simulink library "Vehicle_Visualization"  (R2026a)
settings: Solver=VariableStepAuto
undefined symbols (not defined in the file): unreal_timeseries
libraries: $bdroot x9, sm_car_lib x2, vehdynlibviscommon x1
Description:
  | Copyright 2018-2026 The MathWorks, Inc.
settings Model: Creator=smiller  LastModifiedBy=smiller

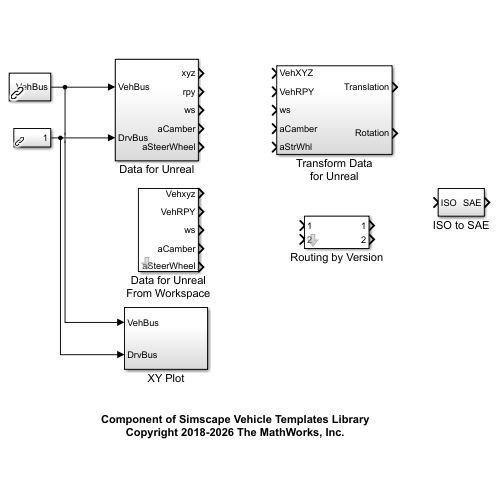
[thumbnail: Simulink's stored preview of the top-level diagram]
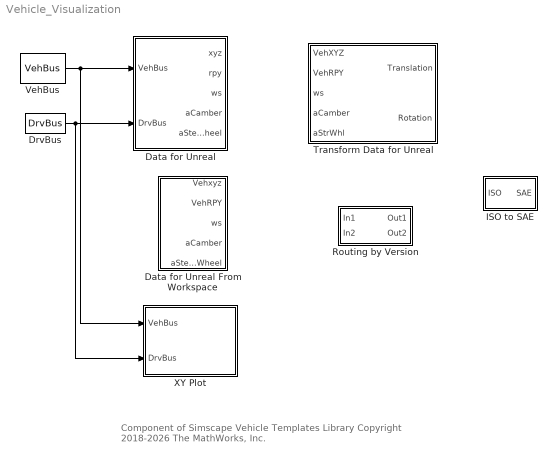
== system Vehicle_Visualization ==
  note: Component of Simscape Vehicle Templates Library
      | Copyright 2018-2026 The MathWorks, Inc.
  Data for Unreal : Subsystem
  Data for Unreal From Workspace : Subsystem  mask(Timeseries data for replay){unreal_data=unreal_timeseries}
      mask prompts: unreal_data "Unreal Time Series"
      mask help: Unpacks timeseries data for use with Vehicle Dynamics Blockset connection to Unreal visualization.
  DrvBus : sm_car_lib/Inputs/DrvBus  SystemSampleTime=-1  VariantActivationTime=update diagram  EmptyChoice=off  PassThrough=off  PassThroughVariantControl=(default)  EmptyChoiceVariantControl=(default)  AllowFlexibleInterface=on  Latency=0  AutoFrameSizeCalculation=off
  ISO to SAE : Subsystem
  Routing by Version : Subsystem  mask(Swap Inputs based on MATLAB Release){post_19a=1}
      mask prompts: post_19a "After R19a?"
      mask help: Unreal Engine inputs of Pitch and Roll were swapped for Wheel Inputs in R2019b. This block swaps order of two inputs based on MATLAB release.
      mask init:
      | if(verLessThan('matlab','9.7'))
      |     set_param(gcb,'post_19a','1');
      | else
      |     set_param(gcb,'post_19a','-1');
      | end
  Transform Data for Unreal : Subsystem
  VehBus : sm_car_lib/Outputs/VehBus  SystemSampleTime=-1  VariantActivationTime=update diagram  EmptyChoice=off  PassThrough=off  PassThroughVariantControl=(default)  EmptyChoiceVariantControl=(default)  AllowFlexibleInterface=on  Latency=0  AutoFrameSizeCalculation=off
  XY Plot : Subsystem
  wires:
  VehBus/1 -> Data for Unreal/1(VehBus), XY Plot/1(VehBus)
  DrvBus/1 -> Data for Unreal/2(DrvBus), XY Plot/2(DrvBus)

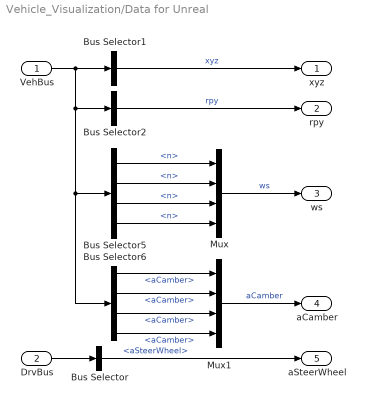
== system Vehicle_Visualization/Data for Unreal ==
  VehBus : Inport
  DrvBus : Inport  Port=2
  Bus Selector : BusSelector  OutputSignals=aSteerWheel
  Bus Selector1 : BusSelector  OutputSignals=World.x,World.y,World.z  OutputAsBus=on
  Bus Selector2 : BusSelector  OutputSignals=World.aRoll,World.aPitch,World.aYaw  OutputAsBus=on
  Bus Selector5 : BusSelector  OutputSignals=Chassis.WhlL1.n,Chassis.WhlR1.n,Chassis.WhlL2.n,Chassis.WhlR2.n
  Bus Selector6 : BusSelector  OutputSignals=Chassis.WhlL1.aCamber,Chassis.WhlR1.aCamber,Chassis.WhlL2.aCamber,Chassis.WhlR2.aCamber
  Mux : Mux
  Mux1 : Mux
  xyz : Outport  VectorParamsAs1DForOutWhenUnconnected=off
  rpy : Outport  Port=2  VectorParamsAs1DForOutWhenUnconnected=off
  ws : Outport  Port=3  VectorParamsAs1DForOutWhenUnconnected=off
  aCamber : Outport  Port=4  VectorParamsAs1DForOutWhenUnconnected=off
  aSteerWheel : Outport  Port=5  VectorParamsAs1DForOutWhenUnconnected=off
  wires:
  Bus Selector5/3 -> Mux/3  "<n>"
  Bus Selector1/1 -> xyz/1  "xyz"
  Mux1/1 -> aCamber/1  "aCamber"
  VehBus/1 -> Bus Selector6/1, Bus Selector5/1, Bus Selector2/1, Bus Selector1/1
  DrvBus/1 -> Bus Selector/1
  Bus Selector5/4 -> Mux/4  "<n>"
  Bus Selector5/2 -> Mux/2  "<n>"
  Bus Selector5/1 -> Mux/1  "<n>"
  Bus Selector6/1 -> Mux1/1  "<aCamber>"
  Bus Selector2/1 -> rpy/1  "rpy"
  Mux/1 -> ws/1  "ws"
  Bus Selector6/2 -> Mux1/2  "<aCamber>"
  Bus Selector6/3 -> Mux1/3  "<aCamber>"
  Bus Selector6/4 -> Mux1/4  "<aCamber>"
  Bus Selector/1 -> aSteerWheel/1  "<aSteerWheel>"

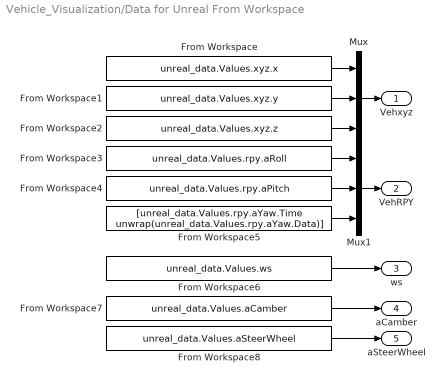
== system Vehicle_Visualization/Data for Unreal From Workspace ==
  From Workspace : FromWorkspace  VariableName=unreal_data.Values.xyz.x
  From Workspace1 : FromWorkspace  VariableName=unreal_data.Values.xyz.y
  From Workspace2 : FromWorkspace  VariableName=unreal_data.Values.xyz.z
  From Workspace3 : FromWorkspace  VariableName=unreal_data.Values.rpy.aRoll
  From Workspace4 : FromWorkspace  VariableName=unreal_data.Values.rpy.aPitch
  From Workspace5 : FromWorkspace  VariableName=[unreal_data.Values.rpy.aYaw.Time unwrap(unreal_data.Values.rpy.aYaw.Data)]
  From Workspace6 : FromWorkspace  VariableName=unreal_data.Values.ws
  From Workspace7 : FromWorkspace  VariableName=unreal_data.Values.aCamber
  From Workspace8 : FromWorkspace  VariableName=unreal_data.Values.aSteerWheel
  Mux : Mux  Inputs=3
  Mux1 : Mux  Inputs=3
  Vehxyz : Outport  VectorParamsAs1DForOutWhenUnconnected=off
  VehRPY : Outport  Port=2  VectorParamsAs1DForOutWhenUnconnected=off
  ws : Outport  Port=3  VectorParamsAs1DForOutWhenUnconnected=off
  aCamber : Outport  Port=4  VectorParamsAs1DForOutWhenUnconnected=off
  aSteerWheel : Outport  Port=5  VectorParamsAs1DForOutWhenUnconnected=off
  wires:
  From Workspace7/1 -> aCamber/1
  From Workspace8/1 -> aSteerWheel/1
  Mux1/1 -> VehRPY/1
  From Workspace3/1 -> Mux1/1
  From Workspace1/1 -> Mux/2
  From Workspace2/1 -> Mux/3
  From Workspace5/1 -> Mux1/3
  From Workspace4/1 -> Mux1/2
  From Workspace6/1 -> ws/1
  Mux/1 -> Vehxyz/1
  From Workspace/1 -> Mux/1

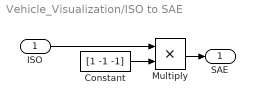
== system Vehicle_Visualization/ISO to SAE ==
  ISO : Inport
  Constant : Constant  Value=[1 -1 -1]
  Multiply : Product
  SAE : Outport  VectorParamsAs1DForOutWhenUnconnected=off
  wires:
  Constant/1 -> Multiply/2
  ISO/1 -> Multiply/1
  Multiply/1 -> SAE/1

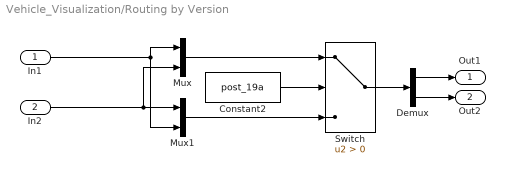
== system Vehicle_Visualization/Routing by Version ==
  In1 : Inport
  In2 : Inport  Port=2
  Constant2 : Constant  Value=post_19a
  Demux : Demux  Outputs=2
  Mux : Mux  Inputs=2
  Mux1 : Mux  Inputs=2
  Switch : Switch  Criteria=u2 > Threshold  SaturateOnIntegerOverflow=off  InputSameDT=off
  Out1 : Outport  VectorParamsAs1DForOutWhenUnconnected=off
  Out2 : Outport  Port=2  VectorParamsAs1DForOutWhenUnconnected=off
  wires:
  Demux/2 -> Out2/1
  Demux/1 -> Out1/1
  Mux1/1 -> Switch/3
  Constant2/1 -> Switch/2
  In1/1 -> Mux1/2, Mux/1
  In2/1 -> Mux1/1, Mux/2
  Mux/1 -> Switch/1
  Switch/1 -> Demux/1

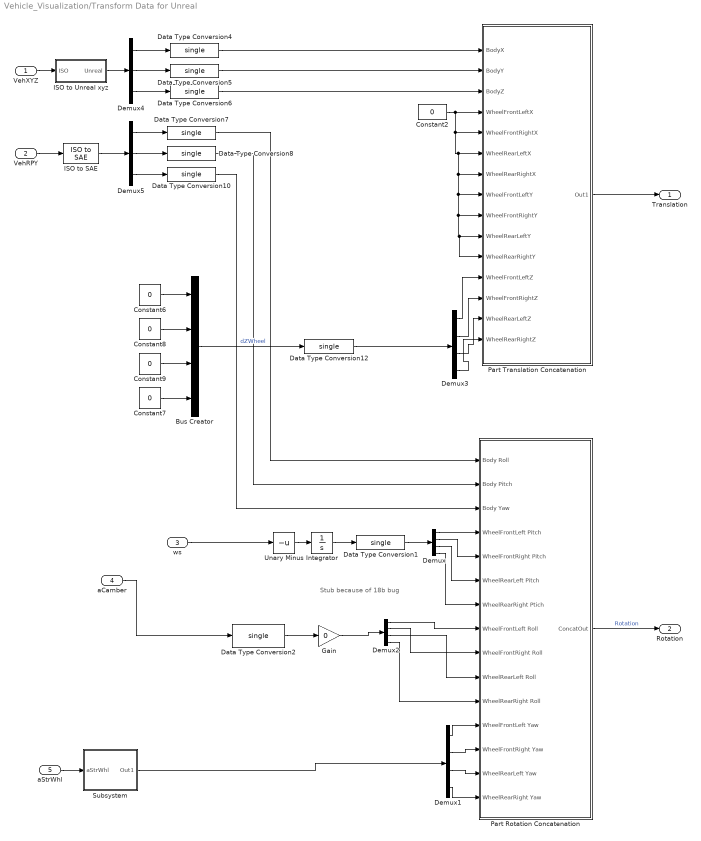
== system Vehicle_Visualization/Transform Data for Unreal ==
  note: Stub because of 18b bug
  VehXYZ : Inport
  VehRPY : Inport  Port=2
  ws : Inport  Port=3
  aCamber : Inport  Port=4
  aStrWhl : Inport  Port=5
  Bus Creator : BusCreator  Inputs=4
  Constant2 : Constant  Value=0  OutDataTypeStr=single
  Constant{6..9} (4 alike) : Constant  Value=0
  Data Type Conversion{1..2,4..8,10,12} (9 alike) : DataTypeConversion  OutDataTypeStr=single  SaturateOnIntegerOverflow=off  RndMeth=Floor
  Demux{,1..3} (4 alike) : Demux
  Demux4 : Demux  Outputs=3
  Demux5 : Demux  Outputs=3
  Gain : Gain  Gain=0
  "ISO to SAE " : $bdroot/ISO to SAE  SystemSampleTime=-1  VariantActivationTime=update diagram  EmptyChoice=off  PassThrough=off  PassThroughVariantControl=(default)  EmptyChoiceVariantControl=(default)  AllowFlexibleInterface=on  Latency=0  AutoFrameSizeCalculation=off
  ISO to Unreal xyz : Subsystem
  Integrator : Integrator
  Part Rotation Concatenation : Subsystem
  Part Translation Concatenation : Subsystem
  Subsystem : Subsystem
  Unary Minus : UnaryMinus
  Translation : Outport  VectorParamsAs1DForOutWhenUnconnected=off
  Rotation : Outport  Port=2  VectorParamsAs1DForOutWhenUnconnected=off
  wires:
  aStrWhl/1 -> Subsystem/1(aStrWhl)
  Part Translation Concatenation/1(Out1) -> Translation/1
  aCamber/1 -> Data Type Conversion2/1
  ws/1 -> Unary Minus/1
  VehRPY/1 -> "ISO to SAE "/1
  "ISO to SAE "/1 -> Demux5/1
  Demux4/2 -> Data Type Conversion5/1
  Demux4/1 -> Data Type Conversion4/1
  ISO to Unreal xyz/1(Unreal) -> Demux4/1
  VehXYZ/1 -> ISO to Unreal xyz/1(ISO)
  Part Rotation Concatenation/1(ConcatOut) -> Rotation/1  "Rotation"
  Subsystem/1(Out1) -> Demux1/1
  Data Type Conversion10/1 -> Part Rotation Concatenation/3(Body Yaw)
  Demux/1 -> Part Rotation Concatenation/4(WheelFrontLeft Pitch)
  Integrator/1 -> Data Type Conversion1/1
  Data Type Conversion2/1 -> Gain/1
  Demux/3 -> Part Rotation Concatenation/6(WheelRearLeft Pitch)
  Demux2/3 -> Part Rotation Concatenation/10(WheelRearLeft Roll)
  Constant7/1 -> Bus Creator/4
  Data Type Conversion6/1 -> Part Translation Concatenation/3(BodyZ)
  Data Type Conversion8/1 -> Part Rotation Concatenation/2(Body Pitch)
  Demux2/1 -> Part Rotation Concatenation/8(WheelFrontLeft Roll)
  Demux2/4 -> Part Rotation Concatenation/11(WheelRearRight Roll)
  Constant6/1 -> Bus Creator/1
  Demux1/2 -> Part Rotation Concatenation/13(WheelFrontRight Yaw)
  Data Type Conversion5/1 -> Part Translation Concatenation/2(BodyY)
  Demux/4 -> Part Rotation Concatenation/7(WheelRearRight Ptich)
  Unary Minus/1 -> Integrator/1
  Constant8/1 -> Bus Creator/2
  Demux1/4 -> Part Rotation Concatenation/15(WheelRearRight Yaw)
  Data Type Conversion1/1 -> Demux/1
  Demux5/1 -> Data Type Conversion7/1
  Demux2/2 -> Part Rotation Concatenation/9(WheelFrontRight Roll)
  Demux1/1 -> Part Rotation Concatenation/12(WheelFrontLeft Yaw)
  Gain/1 -> Demux2/1
  Demux4/3 -> Data Type Conversion6/1
  Data Type Conversion4/1 -> Part Translation Concatenation/1(BodyX)
  Demux5/2 -> Data Type Conversion8/1
  Demux/2 -> Part Rotation Concatenation/5(WheelFrontRight Pitch)
  Demux3/2 -> Part Translation Concatenation/13(WheelFrontRightZ)
  Constant9/1 -> Bus Creator/3
  Demux3/3 -> Part Translation Concatenation/14(WheelRearLeftZ)
  Data Type Conversion12/1 -> Demux3/1
  Demux5/3 -> Data Type Conversion10/1
  Demux3/4 -> Part Translation Concatenation/15(WheelRearRightZ)
  Bus Creator/1 -> Data Type Conversion12/1  "dZWheel"
  Demux3/1 -> Part Translation Concatenation/12(WheelFrontLeftZ)
  Demux1/3 -> Part Rotation Concatenation/14(WheelRearLeft Yaw)
  Constant2/1 -> Part Translation Concatenation/10(WheelRearLeftY), Part Translation Concatenation/11(WheelRearRightY), Part Translation Concatenation/9(WheelFrontRightY), Part Translation Concatenation/8(WheelFrontLeftY), Part Translation Concatenation/7(WheelRearRightX), Part Translation Concatenation/6(WheelRearLeftX), Part Translation Concatenation/5(WheelFrontRightX), Part Translation Concatenation/4(WheelFrontLeftX)
  Data Type Conversion7/1 -> Part Rotation Concatenation/1(Body Roll)

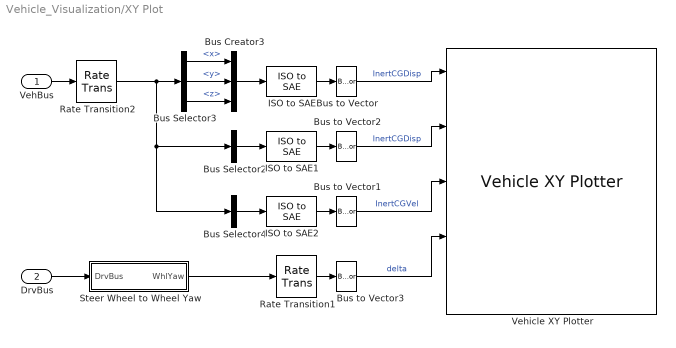
== system Vehicle_Visualization/XY Plot ==
  VehBus : Inport
  DrvBus : Inport  Port=2
  Bus Creator3 : BusCreator  Inputs=3
  Bus Selector2 : BusSelector  OutputSignals=World.aRoll,World.aPitch,World.aYaw  OutputAsBus=on
  Bus Selector3 : BusSelector  OutputSignals=World.x,World.y,World.z
  Bus Selector4 : BusSelector  OutputSignals=World.vx,World.vy,World.vz  OutputAsBus=on
  Bus to Vector{,1..3} (4 alike) : BusToVector
  ISO to SAE : $bdroot/ISO to SAE  SystemSampleTime=-1  VariantActivationTime=update diagram  EmptyChoice=off  PassThrough=off  PassThroughVariantControl=(default)  EmptyChoiceVariantControl=(default)  AllowFlexibleInterface=on  Latency=0  AutoFrameSizeCalculation=off
  ISO to SAE1 : $bdroot/ISO to SAE  SystemSampleTime=-1  VariantActivationTime=update diagram  EmptyChoice=off  PassThrough=off  PassThroughVariantControl=(default)  EmptyChoiceVariantControl=(default)  AllowFlexibleInterface=on  Latency=0  AutoFrameSizeCalculation=off
  ISO to SAE2 : $bdroot/ISO to SAE  SystemSampleTime=-1  VariantActivationTime=update diagram  EmptyChoice=off  PassThrough=off  PassThroughVariantControl=(default)  EmptyChoiceVariantControl=(default)  AllowFlexibleInterface=on  Latency=0  AutoFrameSizeCalculation=off
  Rate Transition1 : RateTransition  Deterministic=off  OutPortSampleTime=0.1
  Rate Transition2 : RateTransition  Deterministic=off  OutPortSampleTime=0.1
  Steer Wheel to Wheel Yaw : Subsystem
  Vehicle XY Plotter : vehdynlibviscommon/Vehicle XY Plotter  w=1.92  a=1.515  b=1.515  tireFMin=tireFMin  figBorder=10  bufferSize=1024  extStats=off  extTireF=off
  wires:
  Rate Transition2/1 -> Bus Selector3/1, Bus Selector4/1, Bus Selector2/1
  Bus Selector2/1 -> ISO to SAE1/1
  Bus to Vector/1 -> Vehicle XY Plotter/1  "InertCGDisp"
  Bus Selector3/2 -> Bus Creator3/2  "<y>"
  Steer Wheel to Wheel Yaw/1(WhlYaw) -> Rate Transition1/1
  Bus to Vector3/1 -> Vehicle XY Plotter/4  "delta"
  VehBus/1 -> Rate Transition2/1
  Bus Selector3/3 -> Bus Creator3/3  "<z>"
  Rate Transition1/1 -> Bus to Vector3/1
  Bus Creator3/1 -> ISO to SAE/1
  Bus Selector4/1 -> ISO to SAE2/1
  Bus Selector3/1 -> Bus Creator3/1  "<x>"
  Bus to Vector1/1 -> Vehicle XY Plotter/3  "InertCGVel"
  Bus to Vector2/1 -> Vehicle XY Plotter/2  "InertCGDisp"
  DrvBus/1 -> Steer Wheel to Wheel Yaw/1(DrvBus)
  ISO to SAE/1 -> Bus to Vector/1
  ISO to SAE1/1 -> Bus to Vector2/1
  ISO to SAE2/1 -> Bus to Vector1/1

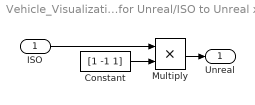
== system Vehicle_Visualization/Transform Data for Unreal/ISO to Unreal xyz ==
  ISO : Inport
  Constant : Constant  Value=[1 -1 1]
  Multiply : Product
  Unreal : Outport  VectorParamsAs1DForOutWhenUnconnected=off
  wires:
  Constant/1 -> Multiply/2
  ISO/1 -> Multiply/1
  Multiply/1 -> Unreal/1

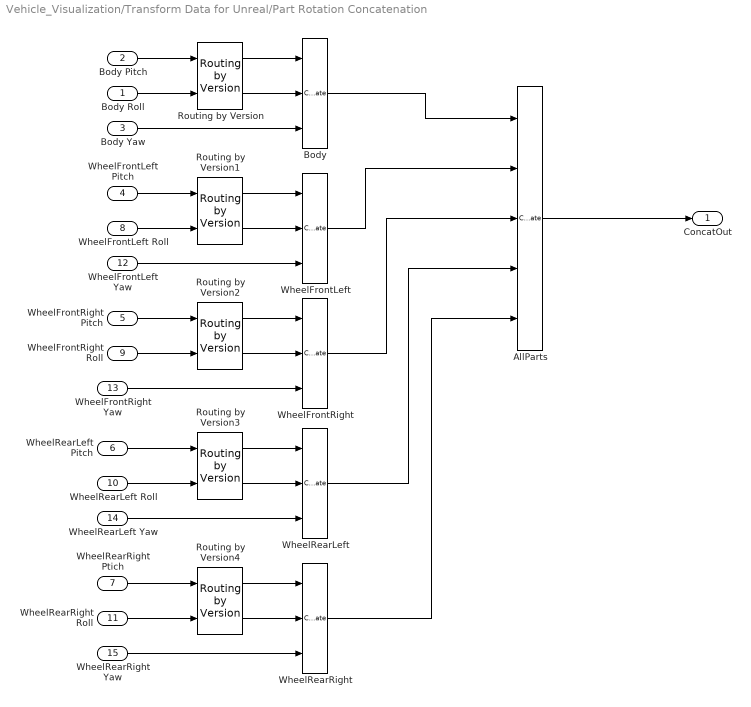
== system Vehicle_Visualization/Transform Data for Unreal/Part Rotation Concatenation ==
  Body Roll : Inport
  Body Pitch : Inport  Port=2
  Body Yaw : Inport  Port=3
  WheelFrontLeft Pitch : Inport  Port=4
  WheelFrontRight Pitch : Inport  Port=5
  WheelRearLeft Pitch : Inport  Port=6
  WheelRearRight Ptich : Inport  Port=7
  WheelFrontLeft Roll : Inport  Port=8
  WheelFrontRight Roll : Inport  Port=9
  WheelRearLeft Roll : Inport  Port=10
  WheelRearRight Roll : Inport  Port=11
  WheelFrontLeft Yaw : Inport  Port=12
  WheelFrontRight Yaw : Inport  Port=13
  WheelRearLeft Yaw : Inport  Port=14
  WheelRearRight Yaw : Inport  Port=15
  AllParts : Concatenate  NumInputs=5  Mode=Multidimensional array
  Body : Concatenate  NumInputs=3  Mode=Multidimensional array  ConcatenateDimension=2
  Routing by Version{,1..4} (5 alike) : $bdroot/Routing by Version  post_19a=-1
  WheelFrontLeft : Concatenate  NumInputs=3  Mode=Multidimensional array  ConcatenateDimension=2
  WheelFrontRight : Concatenate  NumInputs=3  Mode=Multidimensional array  ConcatenateDimension=2
  WheelRearLeft : Concatenate  NumInputs=3  Mode=Multidimensional array  ConcatenateDimension=2
  WheelRearRight : Concatenate  NumInputs=3  Mode=Multidimensional array  ConcatenateDimension=2
  ConcatOut : Outport  VectorParamsAs1DForOutWhenUnconnected=off
  wires:
  Routing by Version4/2 -> WheelRearRight/2
  Routing by Version4/1 -> WheelRearRight/1
  Routing by Version3/2 -> WheelRearLeft/2
  Routing by Version3/1 -> WheelRearLeft/1
  Routing by Version2/2 -> WheelFrontRight/2
  Routing by Version2/1 -> WheelFrontRight/1
  Routing by Version1/2 -> WheelFrontLeft/2
  Routing by Version1/1 -> WheelFrontLeft/1
  Body Pitch/1 -> Routing by Version/1
  Body Roll/1 -> Routing by Version/2
  WheelRearLeft Pitch/1 -> Routing by Version3/1
  WheelFrontRight Pitch/1 -> Routing by Version2/1
  AllParts/1 -> ConcatOut/1
  WheelRearLeft Roll/1 -> Routing by Version3/2
  WheelFrontLeft Roll/1 -> Routing by Version1/2
  WheelFrontRight/1 -> AllParts/3
  WheelFrontRight Yaw/1 -> WheelFrontRight/3
  WheelRearLeft Yaw/1 -> WheelRearLeft/3
  WheelFrontLeft Pitch/1 -> Routing by Version1/1
  Routing by Version/2 -> Body/2
  Routing by Version/1 -> Body/1
  WheelRearRight Ptich/1 -> Routing by Version4/1
  WheelRearRight Yaw/1 -> WheelRearRight/3
  WheelFrontRight Roll/1 -> Routing by Version2/2
  Body/1 -> AllParts/1
  WheelRearLeft/1 -> AllParts/4
  WheelFrontLeft/1 -> AllParts/2
  WheelRearRight Roll/1 -> Routing by Version4/2
  WheelFrontLeft Yaw/1 -> WheelFrontLeft/3
  WheelRearRight/1 -> AllParts/5
  Body Yaw/1 -> Body/3

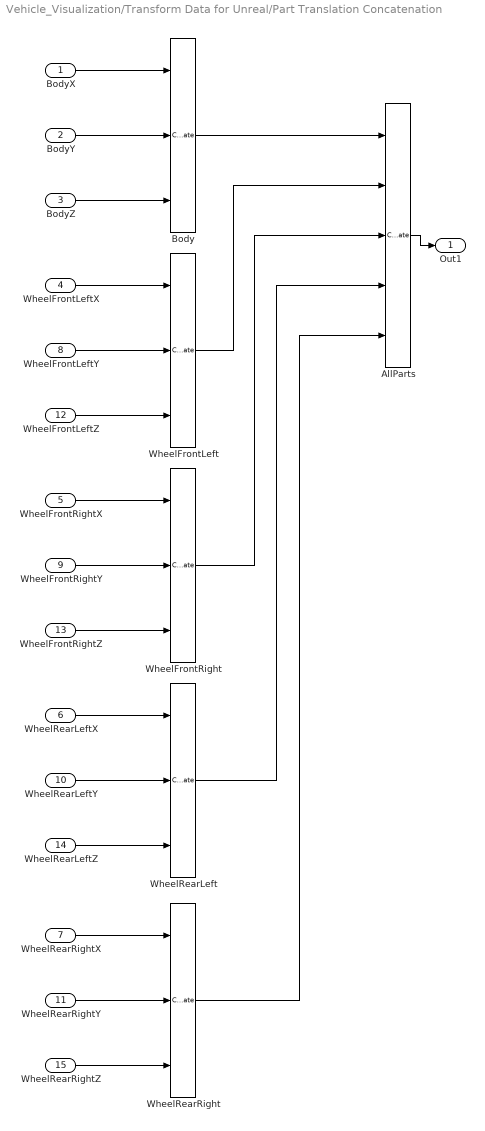
== system Vehicle_Visualization/Transform Data for Unreal/Part Translation Concatenation ==
  BodyX : Inport
  BodyY : Inport  Port=2
  BodyZ : Inport  Port=3
  WheelFrontLeftX : Inport  Port=4
  WheelFrontRightX : Inport  Port=5
  WheelRearLeftX : Inport  Port=6
  WheelRearRightX : Inport  Port=7
  WheelFrontLeftY : Inport  Port=8
  WheelFrontRightY : Inport  Port=9
  WheelRearLeftY : Inport  Port=10
  WheelRearRightY : Inport  Port=11
  WheelFrontLeftZ : Inport  Port=12
  WheelFrontRightZ : Inport  Port=13
  WheelRearLeftZ : Inport  Port=14
  WheelRearRightZ : Inport  Port=15
  AllParts : Concatenate  NumInputs=5  Mode=Multidimensional array
  Body : Concatenate  NumInputs=3  Mode=Multidimensional array  ConcatenateDimension=2
  WheelFrontLeft : Concatenate  NumInputs=3  Mode=Multidimensional array  ConcatenateDimension=2
  WheelFrontRight : Concatenate  NumInputs=3  Mode=Multidimensional array  ConcatenateDimension=2
  WheelRearLeft : Concatenate  NumInputs=3  Mode=Multidimensional array  ConcatenateDimension=2
  WheelRearRight : Concatenate  NumInputs=3  Mode=Multidimensional array  ConcatenateDimension=2
  Out1 : Outport  VectorParamsAs1DForOutWhenUnconnected=off
  wires:
  WheelFrontLeft/1 -> AllParts/2
  WheelFrontRightZ/1 -> WheelFrontRight/3
  WheelFrontRightY/1 -> WheelFrontRight/2
  WheelRearLeftY/1 -> WheelRearLeft/2
  WheelRearRightZ/1 -> WheelRearRight/3
  WheelRearLeftZ/1 -> WheelRearLeft/3
  Body/1 -> AllParts/1
  WheelFrontLeftZ/1 -> WheelFrontLeft/3
  BodyZ/1 -> Body/3
  WheelRearRightX/1 -> WheelRearRight/1
  WheelFrontRight/1 -> AllParts/3
  WheelFrontLeftY/1 -> WheelFrontLeft/2
  WheelRearRightY/1 -> WheelRearRight/2
  WheelRearRight/1 -> AllParts/5
  WheelFrontRightX/1 -> WheelFrontRight/1
  WheelRearLeft/1 -> AllParts/4
  WheelFrontLeftX/1 -> WheelFrontLeft/1
  BodyY/1 -> Body/2
  WheelRearLeftX/1 -> WheelRearLeft/1
  BodyX/1 -> Body/1
  AllParts/1 -> Out1/1

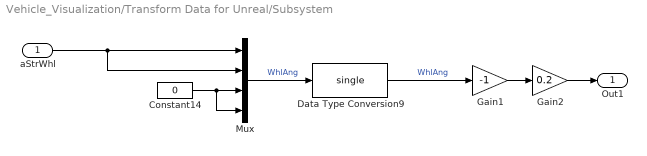
== system Vehicle_Visualization/Transform Data for Unreal/Subsystem ==
  aStrWhl : Inport
  Constant14 : Constant  Value=0
  Data Type Conversion9 : DataTypeConversion  OutDataTypeStr=single  SaturateOnIntegerOverflow=off  RndMeth=Floor
  Gain1 : Gain  Gain=-1
  Gain2 : Gain  Gain=0.2
  Mux : Mux
  Out1 : Outport  VectorParamsAs1DForOutWhenUnconnected=off
  wires:
  Gain2/1 -> Out1/1
  Constant14/1 -> Mux/3, Mux/4
  Mux/1 -> Data Type Conversion9/1  "WhlAng"
  aStrWhl/1 -> Mux/1, Mux/2
  Data Type Conversion9/1 -> Gain1/1  "WhlAng"
  Gain1/1 -> Gain2/1

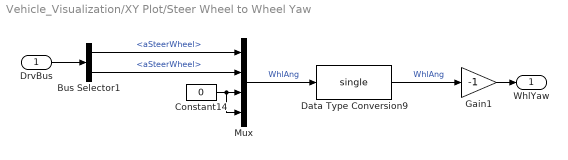
== system Vehicle_Visualization/XY Plot/Steer Wheel to Wheel Yaw ==
  DrvBus : Inport
  Bus Selector1 : BusSelector  OutputSignals=aSteerWheel,aSteerWheel
  Constant14 : Constant  Value=0
  Data Type Conversion9 : DataTypeConversion  OutDataTypeStr=single  SaturateOnIntegerOverflow=off  RndMeth=Floor
  Gain1 : Gain  Gain=-1
  Mux : Mux
  WhlYaw : Outport  VectorParamsAs1DForOutWhenUnconnected=off
  wires:
  Constant14/1 -> Mux/4, Mux/3
  Mux/1 -> Data Type Conversion9/1  "WhlAng"
  Bus Selector1/2 -> Mux/2  "<aSteerWheel>"
  DrvBus/1 -> Bus Selector1/1
  Data Type Conversion9/1 -> Gain1/1  "WhlAng"
  Bus Selector1/1 -> Mux/1  "<aSteerWheel>"
  Gain1/1 -> WhlYaw/1
